simulink model "fwv_fulatti"  (R2021b)
settings: Solver=ode15s  StartTime=0.0  StopTime=10  FixedStep=0.01  MaxStep=0.01  RelTol=1e-3  AbsTol=1e-3  EnableMultiTasking=on
model workspace (MATLAB code in the model file):
  | p0=[0 0 0];
values from neighbouring files (symbols this model uses):
  A_D = 1.5    [main.m]    (also in param.m; params.m)
  A_L = 1.8    [main.m]    (also in param.m; params.m)
  c_bar = S/R    (= 0.0357142857143)    [main.m]    (also in param.m = 0.0251327412287; params.m)
  C_D0 = 0.45    [main.m]    (also in param.m; params.m)
  m = 2    [rbf_pid.m]
  r00 = double(int(f,[0,1]))    [main.m]    (also in param.m = 1; params.m = 0.933333333333)
  r11 = double(int(x*f,[0,1]))    [main.m]    (also in param.m = double(int(curv(x)*(x+1/9),0,1)); params.m = 0.481185185185)
  r22 = double(int(x^2*f,[0,1]))    [main.m]    (also in param.m = double(int(curv(x)*(x+1/9)^2,0,1)); params.m = 0.304750617284)
  r33 = double(int(x^3*f,[0,1]))    [main.m]    (also in param.m = double(int(curv(x)*(x+1/9)^3,0,1)); params.m = 0.218568691358)
  r_cp = Rw*r33/r22    [main.m]    (also in param.m; params.m = 0.10758076225)
  rho = 1.205    [main.m]    (also in param.m; params.m)
  Rw = 0.15    [main.m]    (also in param.m = 0.075; params.m)
  z00 = double(int(f^2,[0,1]))    [main.m]    (also in param.m = double(int(curv(x)^2,0,1)); params.m = 1.00177777778)
  z11 = double(int(x*f^2,[0,1]))    [main.m]    (also in param.m = double(int(curv(x)^2*(x+1/9),0,1)); params.m = 0.484918518519)
  z22 = double(int(x^2*f^2,[0,1]))    [main.m]    (also in param.m = double(int(curv(x)^2*(x+1/9)^2,0,1)); params.m = 0.28785382716)
  zrd = double(int(f^4,[0,1]))    [main.m]    (also in param.m = double(int(curv(x)^4,0,1)); params.m = 1.29333866667)
undefined symbols (not defined in the file or in its folder): X, Y, Z
libraries: sm_lib x57, nesl_utility x45, vrlib x3, slpidlib x2
(part 1 of 3)
settings Model: NumberOfSteps=10  PacingRate=1000  Creator=jeff  LastModifiedBy=jeff
settings SolverCC: AutoScaleAbsTol=off  ZeroCrossAlgorithm=Adaptive  SolverResetMethod=Robust
settings DataIOCC: LimitDataPoints=on  MaxDataPoints=10000  DSMLogging=off  InspectSignalLogs=on  SaveTime=off  ReturnWorkspaceOutputs=off
settings OptimizationCC: LifeSpan=inf
settings DebuggingCC: AllowSymbolicDim=off  SFUnexpectedBacktrackingDiag=warning  SFNoUnconditionalDefaultTransitionDiag=warning  SFExecutionAtInitializationDiag=none  SFMachineParentedDataDiag=warning  ArithmeticOperatorsInVariantConditions=warning
settings ModelReferenceCC: ModelReferenceMinAlgLoopOccurrences=on
settings SFSimCC: SimUseLocalCustomCode=off  CustomCodeUndefinedFunction=UseInterfaceOnly
settings RTWCC: RTWUseLocalCustomCode=off
settings CodeAppCC: StateflowObjectComments=on
settings GRTTargetCC: TargetLangStandard=C89/C90 (ANSI)
settings ConfigComp: CovMetricSettings=dw  CovSaveCumulativeToWorkspaceVar=on  CovSaveSingleToWorkspaceVar=on  CovExternalEMLEnable=off  CovSFcnEnable=off
settings SimscapeCC: SimscapeLogType=all  SimscapeLogSimulationStatistics=on  SimscapeLogDataHistory=10000
settings ExplorerConfigSet: InternalSimMechanicsExplorerSettings="<ExplorerConfiguration><canonicalview>default</canonicalview><AnimationSetting><BasePlaybackSpeed>1.0</BasePlaybackSpeed><PlaybackSpeedFactor>1.0</PlaybackSpeedFactor></AnimationSetting><TilePanel><TileInfo><Tiles Columns=\"2\" Count=\"4\" Rows=\"2\"><Column Weight=\"0.5\"/><Column Weight=\"0.5\"/><Row Weight=\"0.4982\"/><Row Weight=\"0.5018\"/><Tile Height=\"1\" Width=\"1\" X=\"0\" Y=\"0\"/><Tile Height=\"1\" Width=\"1\" X=\"0\" Y=\"1\"/><Tile Height=\"1\" Width=\"1\" X=\"1\" Y=\"0\"/><Tile Height=\"1\" Width=\"1\" X=\"1\" Y=\"1\"/></Tiles></TileInfo><SceneInfo><SceneViewer><BGColor><R>0.60000002384185791</R><G>0.60000002384185791</G><B>0.60000002384185791</B></BGColor><Camera><DoPerspective>off</DoPerspective><Position><X>1.52276591336431011e-07</X><Y>-15.7283506478538051</Y><Z>0.997276938595945239</Z></Position><Center><X>1.52276591336431011e-07</X><Y>8.81149515574719544e-08</Y><Z>0.997276938595945239</Z></Center><Up><X>0</X><Y>-0</Y><Z>1</Z></Up><ViewLimDist>1</ViewLimDist><YLim>4.13867069486404926</YLim><XLim>10.3000000000000007</XLim></Camera></SceneViewer><SceneViewer><BGColor><R>0.60000002384185791</R><G>0.60000002384185791</G><B>0.60000002384185791</B></BGColor><Camera><DoPerspective>off</DoPerspective><Position><X>1.52276591336431011e-07</X><Y>-4.72670020457144346e-07</Y><Z>14.1965844691727394</Z></Position><Center><X>1.52276591336431011e-07</X><Y>-4.72670020457144346e-07</Y><Z>0.997276770136494406</Z></Center><Up><X>0</X><Y>1</Y><Z>-0</Z></Up><ViewLimDist>1</ViewLimDist><YLim>10.3000000000000007</YLim><XLim>25.4425373134328368</XLim></Camera></SceneViewer><SceneViewer><BGColor><R>0.60000002384185791</R><G>0.60000002384185791</G><B>0.60000002384185791</B></BGColor><Camera><DoPerspective>off</DoPerspective><Position><X>15.7283506450403667</X><Y>-4.72670020457144346e-07</Y><Z>0.997277415433075021</Z></Position><Center><X>1.16597679067353965e-06</X><Y>-4.72670020457144346e-07</Y><Z>0.997277415433075021</Z></Center><Up><X>-0</X><Y>0</Y><Z>1</Z></Up><ViewLimDist>1</ViewLimDist><YLim>4.13867069486404926</YLim><XLim>10.3000000000000007</XLim></Camera></SceneViewer><SceneViewer><BGColor><R>0.60000002384185791</R><G>0.60000002384185791</G><B>0.60000002384185791</B></BGColor><Camera><DoPerspective>on</DoPerspective><Position><X>2.15185180954951205</X><Y>2.000061471445302</Y><Z>2.10008566610887026</Z></Position><Center><X>2.00185180954951214</X><Y>2.000061471445302</Y><Z>2.00008566610887017</Z></Center><Up><X>0</X><Y>-3.08148791101957736e-33</Y><Z>1</Z></Up><ViewLimDist>1</ViewLimDist><YLim>0.466307658154998583</YLim><XLim>1.15184951380078004</XLim></Camera></SceneViewer></SceneInfo></TilePanel><MechEditorPanel><Cameras><Camera><Id>Camera1</Id><Value><Name>Camera1</Name><NativeCamera><PositionTrackingFeature>FWV.camera.camera_Frame.R</PositionTrackingFeature><CenterTrackingFeature>FWV.camera.C</CenterTrackingFeature><UpVectorTrackingFeature>FWV.camera.C</UpVectorTrackingFeature><CenterTrackingOrigin>on</CenterTrackingOrigin><UpVectorTrackingDirection>+Z</UpVectorTrackingDirection></NativeCamera></Value></Camera></Cameras><GfxPanelCameraMap><MapElement CameraMLId=\"Camera1\" GfxPanelIndex=\"3\"/></GfxPanelCameraMap><VideoCreator><PlaybackSpeedRatio>1.0</PlaybackSpeedRatio><FrameRate>30</FrameRate><VideoFormat>Motion JPEG AVI</VideoFormat><FrameSize>auto</FrameSize></VideoCreator></MechEditorPanel></ExplorerConfiguration>"

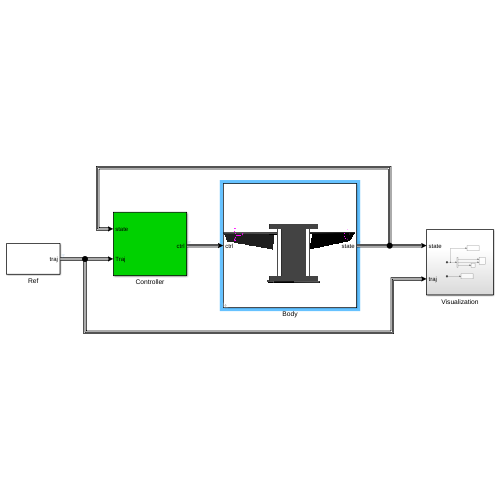
[thumbnail: Simulink's stored preview of the top-level diagram]
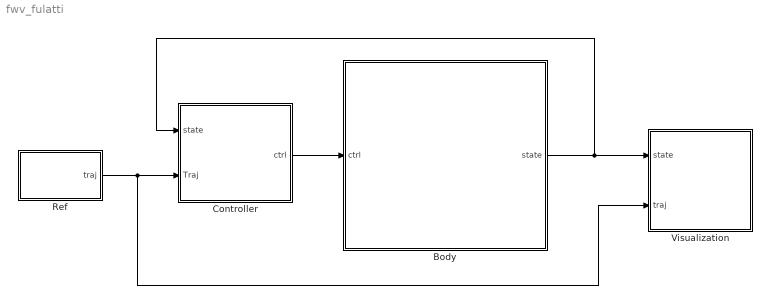
== system fwv_fulatti ==
  Body : Subsystem  mask{rho_w=900, m_t=20, stif_stk=0, stif_rot=5e-3, damp_rot=0, stif_m=1e2, damp_m=1e2, z0=0, p0=0, q0=0, r0=0}
      mask prompts: z0 "initial height"; p0 "initial roll(deg)"; q0 "initial pitch(deg)"; r0 "initial yaw(deg)"
      mask Display: image('Images/fwv.png');
  Controller : Subsystem
  Ref : Subsystem
  Visualization : Subsystem
  wires:
  Ref/1(traj) -> Visualization/2(traj), Controller/2(Traj)
  Controller/1(ctrl) -> Body/1(ctrl)
  Body/1(state) -> Controller/1(state), Visualization/1(state)

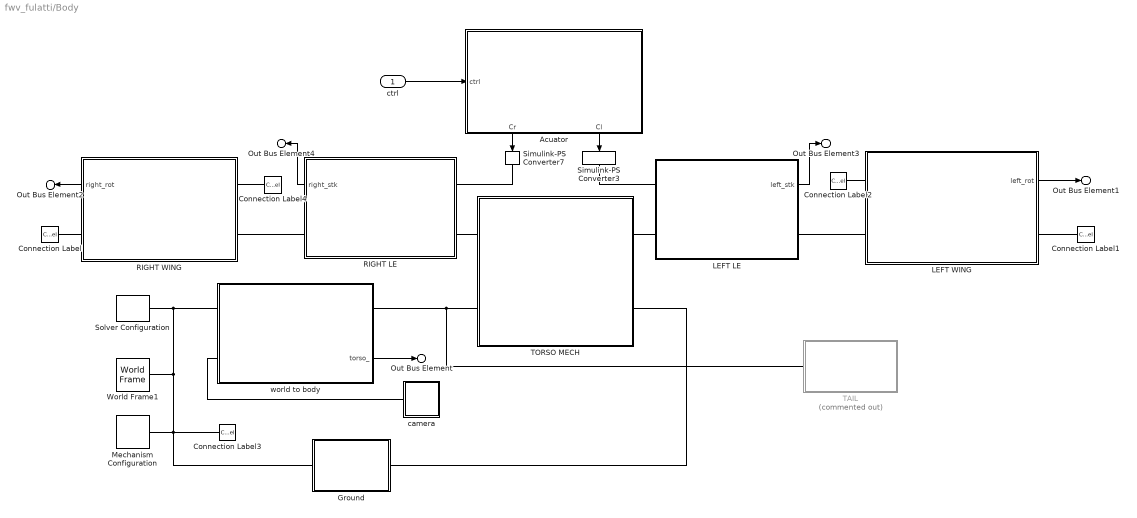
== system fwv_fulatti/Body ==
  ctrl : Inport
  Acuator : Subsystem
      settings: PortSchema="{\"entries\":[{\"content\":{\"sides\":[{\"content\":{\"connectorIds\":[\"In1\"]},\"type\":\"ConnectorPlacement.EquallySpacedRectSide\",\"uuid\":\"db46f0ff-2b35-4735-b2ba-99ebad500531\"},{\"content\":{\"connectorIds\":[],\"side\":\"RIGHT\"},\"type\":\"ConnectorPlacement.EquallySpacedRectSide\",\"uuid\":\"a05d2a9d-5b8e-445a-bb52-abca9ea78047\"},{\"content\":{\"connectorIds\":[],\"side\":\"TOP\"},\"type\":\"ConnectorPlacement.EquallySpacedRectSide\",\"uuid\":\"a9e07a0b-59af-45c6-89e8-be07490c71bb\"},{\"content\":{\"connectorIds\":[\"Out1\",\"Out2\"],\"side\":\"BOTTOM\"},\"type\":\"ConnectorPlacement.EquallySpacedRectSide\",\"uuid\":\"69a70806-995a-45b1-874e-667630f2a15c\"}]},\"type\":\"ConnectorPlacement.EquallySpacedConnector\",\"uuid\":\"cc8e5811-56fa-45cd-8c97-474062c30ea3\"}],\"packageUris\":[\"http://schema.mathworks.com/mf0/Connector/R2020b\"],\"version\":\"1.0\"}"
  Connection Label : ConnectionLabel  Label=CP_R
  Connection Label1 : ConnectionLabel  Label=CP_L
  Connection Label2 : ConnectionLabel  Label=W
  Connection Label3 : ConnectionLabel  Label=W
  Connection Label4 : ConnectionLabel  Label=W
  Ground : Subsystem
  LEFT LE : Subsystem
      mask Display: image('Images/lle.png'); % Use "Edit Image" on toolstrip to change.
  LEFT WING : Subsystem
      mask Display: image('Images/lwing.png'); % Use "Edit Image" on toolstrip to change.
  Mechanism Configuration : sm_lib/Utilities/Mechanism Configuration  UniformGravity=Constant  GravityVector=[0 0 -9.80665]  GravityUnits=m/s^2  LinearizationDelta=0.001  JointModeTransitionNonlinearIterations=2
  RIGHT LE : Subsystem
      settings: PortSchema="{\"entries\":[{\"content\":{\"sides\":[{\"content\":{\"connectorIds\":[\"Out1\",\"LConn1\"]},\"type\":\"ConnectorPlacement.EquallySpacedRectSide\",\"uuid\":\"e80f0529-82a8-4e91-8f70-1f5fff48efb0\"},{\"content\":{\"connectorIds\":[\"RConn1\",\"RConn2\"],\"side\":\"RIGHT\"},\"type\":\"ConnectorPlacement.EquallySpacedRectSide\",\"uuid\":\"c7e3ee7d-7bee-46da-b210-768e5832b89d\"},{\"content\":{\"connectorIds\":[],\"side\":\"TOP\"},\"type\":\"ConnectorPlacement.EquallySpacedRectSide\",\"uuid\":\"680cbd67-40e5-4a58-a196-f2062cf587c7\"}]},\"type\":\"ConnectorPlacement.EquallySpacedConnector\",\"uuid\":\"7cb1a5ec-7352-40bf-9e6c-a29cba360f94\"}],\"packageUris\":[\"http://schema.mathworks.com/mf0/Connector/R2020b\"],\"version\":\"1.0\"}"
      mask Display: image('Images/rle.png'); % Use "Edit Image" on toolstrip to change.
  RIGHT WING : Subsystem
      mask Display: image('Images/rwing.png'); % Use "Edit Image" on toolstrip to change.
  Simulink-PS Converter3 : nesl_utility/Simulink-PS Converter  PhysicalDomain=network_engine_domain  SubClassName=ps_input  LeftPortType=input  RightPortType=output  PseudoPeriodic=off  Frequencies=[]  NoiseDistribution=none  NoiseParameters=[]  Unit=1  AffineConversion=off  FilteringAndDerivatives=filter  SimscapeFilterOrder=2  InputFilterTimeConstant=0.001  UdotUserProvided=2
      settings: SourceProductBaseCode=PW,SS
  Simulink-PS Converter7 : nesl_utility/Simulink-PS Converter  PhysicalDomain=network_engine_domain  SubClassName=ps_input  LeftPortType=input  RightPortType=output  PseudoPeriodic=off  Frequencies=[]  NoiseDistribution=none  NoiseParameters=[]  Unit=1  AffineConversion=off  FilteringAndDerivatives=filter  SimscapeFilterOrder=2  InputFilterTimeConstant=0.001  UdotUserProvided=0
      settings: SourceProductBaseCode=PW,SS
  Solver Configuration : nesl_utility/Solver Configuration  PhysicalDomain=network_engine_domain  SubClassName=solver  LeftPortType=input  RightPortType=generic  Tones=[]  Harmonics=[]  SimulateNoise=off  Profile=off  UseLocalSampling=off  EnableSwitchedLinearOptims=on  FrequencyDomain=off  UseCCode=off  RelTol=0.001  AbsTol=1e-06  MinStep=1e-09  ToWorkspace=off  RevertToSquareIcSolve=off  NumHomotopyIterations=100  PhasorMode=off  PhasorModeNumHarmonics=1  DoDC=off  ResidualTolerance=1e-09  UseLocalSolver=off  LocalSolverChoice=NE_BACKWARD_EULER_ADVANCER  LocalSolverSampleTime=0.001  DoFixedCost=off  MaxNonlinIter=3  MaxModeIter=2  ComputeImpulses=off  ImpulseIterations=2  LinearAlgebra=Sparse  EquationFormulation=NE_TIME_EF  DelaysMemoryBudget=1024  AutomaticFiltering=on  FilteringTimeConstant=0.001  PartitionStorageMethod=AS_NEEDED  PartitionMemoryBudget=1024  PartitionMethod=FAST
      settings: SourceProductBaseCode=PW,SS
  TAIL : Subsystem  Commented=on
  TORSO MECH : Subsystem  mask{mu0=0, mu1=0}
      mask Display: image('Images/fuselage.png'); % Use "Edit Image" on toolstrip to change.
  World Frame1 : sm_lib/Frames and Transforms/World Frame
  camera : Subsystem
  world to body : Subsystem
      settings: PortSchema="{\"entries\":[{\"content\":{\"sides\":[{\"content\":{\"connectorIds\":[\"LConn1\",\"LConn2\"]},\"type\":\"ConnectorPlacement.EquallySpacedRectSide\",\"uuid\":\"67e08b7d-27a7-478e-aa2b-0a29cfb8c4ba\"},{\"content\":{\"connectorIds\":[\"RConn1\",\"Out1\"],\"side\":\"RIGHT\"},\"type\":\"ConnectorPlacement.EquallySpacedRectSide\",\"uuid\":\"af848fd7-c404-4734-a34f-7cffff1411b1\"},{\"content\":{\"connectorIds\":[],\"side\":\"TOP\"},\"type\":\"ConnectorPlacement.EquallySpacedRectSide\",\"uuid\":\"40c86437-2469-4d2e-8b61-7b3eee85e893\"}]},\"type\":\"ConnectorPlacement.EquallySpacedConnector\",\"uuid\":\"cd10b607-3f85-4cd2-a6c3-0d07bf2597bd\"}],\"packageUris\":[\"http://schema.mathworks.com/mf0/Connector/R2020b\"],\"version\":\"1.0\"}"
  Out Bus Element : Outport  PortName=state  Element=pose
  Out Bus Element3 : Outport  PortName=state  Element=left_stk
  Out Bus Element1 : Outport  PortName=state  Element=left_rot
  Out Bus Element4 : Outport  PortName=state  Element=right_stk
  Out Bus Element2 : Outport  PortName=state  Element=right_rot
  wires:
  LEFT WING/1(left_rot) -> Out Bus Element1/1
  RIGHT WING/1(right_rot) -> Out Bus Element2/1
  world to body/1(torso_) -> Out Bus Element/1
  Acuator/2(Cl) -> Simulink-PS Converter3/1
  Acuator/1(Cr) -> Simulink-PS Converter7/1
  ctrl/1 -> Acuator/1(ctrl)
  LEFT LE/1(left_stk) -> Out Bus Element3/1
  RIGHT LE/1(right_stk) -> Out Bus Element4/1
  connections:
  LEFT LE/LConn2 -- TORSO MECH/RConn1
  TORSO MECH/LConn1 -- RIGHT LE/RConn2
  Simulink-PS Converter7/RConn1 -- RIGHT LE/RConn1
  Mechanism Configuration/RConn1 -- Connection Label3/LConn1 -- Ground/LConn1 -- world to body/LConn1 -- Solver Configuration/RConn1 -- World Frame1/RConn1
  world to body/RConn1 -- TAIL/LConn1 -- TORSO MECH/LConn2
  camera/LConn1 -- world to body/LConn2
  Ground/RConn1 -- TORSO MECH/RConn2
  Connection Label/LConn1 -- RIGHT WING/RConn1
  LEFT WING/RConn1 -- Connection Label1/LConn1
  Simulink-PS Converter3/RConn1 -- LEFT LE/LConn1
  LEFT WING/LConn2 -- LEFT LE/RConn1
  RIGHT WING/LConn2 -- RIGHT LE/LConn1
  Connection Label2/LConn1 -- LEFT WING/LConn1
  Connection Label4/LConn1 -- RIGHT WING/LConn1

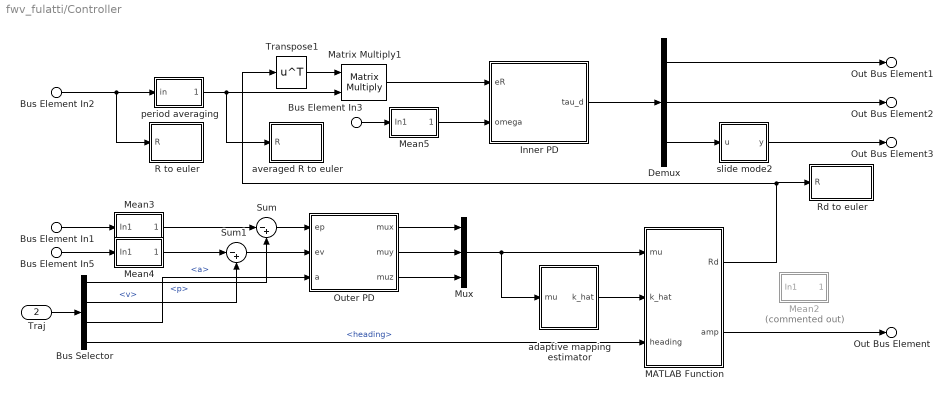
== system fwv_fulatti/Controller ==
  Bus Element In1 : Inport  PortName=state  Element=pose.p
  Bus Element In2 : Inport  PortName=state  Element=pose.R
  Bus Element In3 : Inport  PortName=state  Element=pose.w
  Bus Element In5 : Inport  PortName=state  Element=pose.v
  Traj : Inport  Port=2
  Bus Selector : BusSelector  OutputSignals=p,v,a,heading
  Demux : Demux  Outputs=3
  Inner PD : Subsystem
  MATLAB Function : MATLAB Function  TreatAsAtomicUnit=on
  Matrix Multiply1 : Product  Multiplication=Matrix(*)
  Mean2 : Subsystem  Commented=on
  Mean3 : Subsystem
  Mean4 : Subsystem
  Mean5 : Subsystem
  Mux : Mux  Inputs=3
  Outer PD : Subsystem
  R to euler : Subsystem
  Rd to euler : Subsystem
      settings: PortSchema="{\"entries\":[{\"content\":{\"sides\":[{\"content\":{\"connectorIds\":[]},\"type\":\"ConnectorPlacement.EquallySpacedRectSide\",\"uuid\":\"93de112d-0217-40d7-a336-17ea7cc4ed84\"},{\"content\":{\"connectorIds\":[\"In1\"],\"side\":\"RIGHT\"},\"type\":\"ConnectorPlacement.EquallySpacedRectSide\",\"uuid\":\"0b203bc8-f5c1-4f94-b862-0e0b0c3261f7\"},{\"content\":{\"connectorIds\":[],\"side\":\"TOP\"},\"type\":\"ConnectorPlacement.EquallySpacedRectSide\",\"uuid\":\"1be19d4c-6517-470f-aabd-96bb4bcaed3d\"}]},\"type\":\"ConnectorPlacement.EquallySpacedConnector\",\"uuid\":\"f5fc68b0-193c-43e6-a8c2-776496b24de9\"}],\"packageUris\":[\"http://schema.mathworks.com/mf0/Connector/R2020b\"],\"version\":\"1.0\"}"
  Sum : Sum  Inputs=|-+
  Sum1 : Sum  Inputs=|-+
  Transpose1 : Math  Operator=transpose  SaturateOnIntegerOverflow=on
  adaptive mapping estimator : Subsystem
  averaged R to euler : Subsystem
  period averaging : Subsystem
  slide mode2 : MATLAB Function  TreatAsAtomicUnit=on
  Out Bus Element : Outport  PortName=ctrl  Element=amp_mean
  Out Bus Element1 : Outport  PortName=ctrl  Element=amp_diff
  Out Bus Element2 : Outport  PortName=ctrl  Element=bias
  Out Bus Element3 : Outport  PortName=ctrl  Element=offset
  wires:
  Traj/1 -> Bus Selector/1
  Bus Selector/1 -> Sum/2  "<p>"
  Inner PD/1(tau_d) -> Demux/1
  Transpose1/1 -> Matrix Multiply1/1
  Bus Selector/2 -> Sum1/2  "<v>"
  Bus Selector/3 -> Outer PD/3(a)  "<a>"
  Bus Element In2/1 -> R to euler/1(R), period averaging/1(in)
  Bus Selector/4 -> MATLAB Function/3(heading)  "<heading>"
  Sum/1 -> Outer PD/1(ep)
  Sum1/1 -> Outer PD/2(ev)
  Outer PD/3(muz) -> Mux/3
  Mux/1 -> MATLAB Function/1(mu), adaptive mapping estimator/1(mu)
  Matrix Multiply1/1 -> Inner PD/1(eR)
  Demux/3 -> slide mode2/1(u)
  MATLAB Function/1(Rd) -> Transpose1/1, Rd to euler/1(R)
  Bus Element In1/1 -> Mean3/1(In1)
  Bus Element In5/1 -> Mean4/1(In1)
  Mean3/1(Mean1) -> Sum/1
  Mean4/1(Mean1) -> Sum1/1
  Bus Element In3/1 -> Mean5/1(In1)
  Mean5/1(Mean1) -> Inner PD/2(omega)
  MATLAB Function/2(amp) -> Out Bus Element/1
  period averaging/1(Mean1) -> averaged R to euler/1(R), Matrix Multiply1/2
  adaptive mapping estimator/1(k_hat) -> MATLAB Function/2(k_hat)
  Outer PD/1(mux) -> Mux/1
  Outer PD/2(muy) -> Mux/2
  Demux/1 -> Out Bus Element1/1
  Demux/2 -> Out Bus Element2/1
  slide mode2/1(y) -> Out Bus Element3/1

== system fwv_fulatti/Ref ==
  Bus Creator : BusCreator  Inputs=4
  Clock : Clock
  p,pdot,pddot : MATLAB Function  TreatAsAtomicUnit=on
  traj : Outport
  wires:
  Bus Creator/1 -> traj/1
  p,pdot,pddot/3(v) -> Bus Creator/3  "v"
  p,pdot,pddot/4(a) -> Bus Creator/4  "a"
  Clock/1 -> p,pdot,pddot/1(t)
  p,pdot,pddot/1(p) -> Bus Creator/1  "p"
  p,pdot,pddot/2(heading) -> Bus Creator/2

== system fwv_fulatti/Visualization ==
  Bus Element In1 : Inport  PortName=state  Element=pose.p
  Bus Element In : Inport  Port=2  PortName=traj  Element=p
  Demux : Demux  Outputs=3
  Terminator : Terminator
  To Workspace : ToWorkspace  VariableName=p  SampleTime=-1
      settings: Save2DSignal=2-D array (concatenate along first dimension)
  To Workspace1 : ToWorkspace  VariableName=pd  SampleTime=-1
      settings: Save2DSignal=2-D array (concatenate along first dimension)
  XY Graph : Record  FileSettingsInternal="{\"entries\":[{\"content\":{\"excelSettings\":{\"content\":{},\"type\":\"Streamout.ExcelSettings\"}},\"type\":\"Streamout.FileSettingStorage\",\"uuid\":\"cf1958ac-8bfe-45ed-8e34-609005fdbf73\"}],\"packageUris\":[\"http://schema.mathworks.com/mf0/streamout_blocks/R2020a\"],\"version\":\"1.0\"}"  Layout=[1 1]  SignalsInternal="{\"entries\":[{\"content\":{\"signals\":[{\"content\":{\"blockPath\":[\"fwv_fulatti/Visualization/XY Graph\"],\"channel\":[],\"dimensions\":[1],\"domain\":\"fwv_fulatti/Visualization/XY Graph\",\"lineColor\":\"#fe330a\",\"plots\":[],\"port\":1,\"sid\":[\"\"],\"signalID\":154858,\"signalName\":\"Demux:1\"},\"type\":\"RecordBlkView.Signal\",\"uuid\":\"53ba67ad-0e88-436d-a209-32f50bd88dfe\"},{\"content\":{\"blockPath\":[\"fwv_fulatti/Visualization/XY Graph\"],\"channel\":[],\"dimensions\":[1],\"domain\":\"fwv_fulatti/Visualization/XY Graph\",\"lineColor\":\"#22b573\",\"plots\":[],\"port\":2,\"sid\":[\"\"],\"signalID\":154862,\"signalName\":\"Demux:2\"},\"type\":\"RecordBlkView.Signal\",\"uuid\":\"95253e4f-1692-44e6-a8ad-d105dc3e908e\"}]},\"type\":\"RecordBlkView.InputSignals\",\"uuid\":\"3e219576-be3c-4ed1-8d49-ea9d7e7a7c36\"}],\"packageUris\":[\"http://schema.mathworks.com/mf0/streamout_blocks/R2020a\"],\"version\":\"1.0\"}"  VisualizationBindings="{\"xyplotplugin\":{\"info\":[{\"series\":[],\"subplotID\":1}]}}"  CompatibilityTag=XY  st=-1
  wires:
  Bus Element In1/1 -> To Workspace/1, Demux/1
  Demux/3 -> Terminator/1
  Demux/1 -> XY Graph/1
  Demux/2 -> XY Graph/2
  Bus Element In/1 -> To Workspace1/1

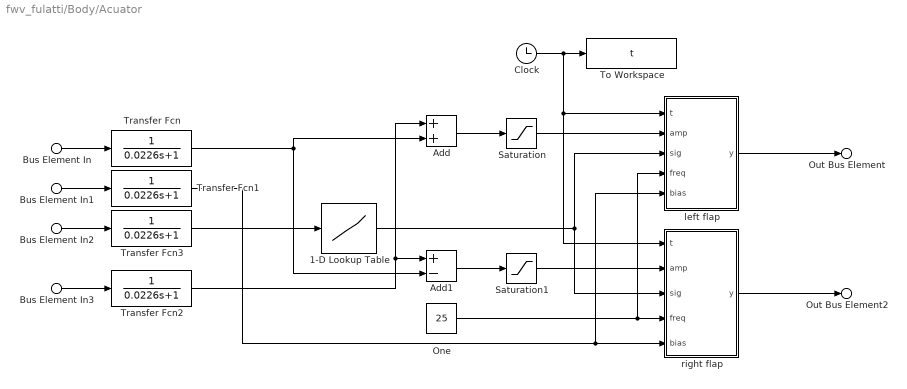
== system fwv_fulatti/Body/Acuator ==
  Bus Element In3 : Inport  PortName=ctrl  Element=amp_mean
  Bus Element In : Inport  PortName=ctrl  Element=amp_diff
  Bus Element In1 : Inport  PortName=ctrl  Element=bias
  Bus Element In2 : Inport  PortName=ctrl  Element=offset
  " left flap" : MATLAB Function  TreatAsAtomicUnit=on
  " right flap" : MATLAB Function  TreatAsAtomicUnit=on
  1-D Lookup Table : Lookup_n-D  NumberOfTableDimensions=1  BreakpointsForDimension1=[-1:1]  Table=1.0./(1+exp(-10*[-1:1]))  InternalRulePriority=Speed  RndMeth=Simplest  InputSameDT=on
  Add : Sum
  Add1 : Sum  Inputs=+-
  Clock : Clock
  One : Constant  Value=25  OutDataTypeStr=Inherit: Inherit via back propagation
  Saturation : Saturate  UpperLimit=pi/2  LowerLimit=0  ZeroCross=off
  Saturation1 : Saturate  UpperLimit=pi/2  LowerLimit=0  ZeroCross=off
  To Workspace : ToWorkspace  VariableName=t  SampleTime=-1
  Transfer Fcn{,1..3} (4 alike) : TransferFcn  Denominator=[0.0226 1]
  Out Bus Element2 : Outport  PortName=Cr  Element=stroke
  Out Bus Element : Outport  Port=2  PortName=Cl  Element=stroke
  wires:
  Add1/1 -> Saturation1/1
  " left flap"/1(y) -> Out Bus Element/1
  One/1 -> " left flap"/4(freq), " right flap"/4(freq)
  " right flap"/1(y) -> Out Bus Element2/1
  Add/1 -> Saturation/1
  Saturation/1 -> " left flap"/2(amp)
  Clock/1 -> " right flap"/1(t), " left flap"/1(t), To Workspace/1
  Saturation1/1 -> " right flap"/2(amp)
  Transfer Fcn2/1 -> Add/1, Add1/1
  Transfer Fcn/1 -> Add1/2, Add/2
  Bus Element In/1 -> Transfer Fcn/1
  Bus Element In1/1 -> Transfer Fcn1/1
  Bus Element In2/1 -> Transfer Fcn3/1
  Bus Element In3/1 -> Transfer Fcn2/1
  Transfer Fcn1/1 -> " left flap"/5(bias), " right flap"/5(bias)
  Transfer Fcn3/1 -> 1-D Lookup Table/1
  1-D Lookup Table/1 -> " right flap"/3(sig), " left flap"/3(sig)

== system fwv_fulatti/Body/Ground ==
  Cylindrical Solid : sm_lib/Body Elements/Cylindrical Solid  GraphicAmbientColor=[0.15 0.15 0.15 1.0]  BasedOnType=Mass  CenterOfMass=[0 0 0]  CenterOfMassUnits=m  GraphicDiffuseColor=[1.0 0.2 0.4]  CylinderLength=1  CylinderLengthUnits=mm  CylinderRadius=10  CylinderRadiusUnits=m  Density=1000  DensityUnits=kg/m^3  DoExposeReferenceFrame=off  GraphicEmissiveColor=[0.0 0.0 0.0 1.0]  ExportEntireGeometry=on  SerializedFrames=<Frames><Frame><Id>Frame1</Id><Value><Name>F1</Name><Origin><Source>GeometricFeature</Source><FeatureName>top surface</FeatureName></Origin><PrimaryAxis><DefinedDirection>+Z</DefinedDirection><Source>ReferenceFrame</Source><SourceDirection>+Z</SourceDirection><FeatureName></FeatureName></PrimaryAxis><SecondaryAxis><DefinedDirection>+X</DefinedDirection><Source>ReferenceFrame</Source><SourceDirection>+X</SourceDirection><FeatureName></FeatureName></SecondaryAxis></Value></Frame></Frames>  MarkerShape=Sphere  MarkerSize=10  GraphicType=FromGeometry  InertiaType=Custom  Mass=0  MassUnits=kg  MomentsOfInertia=[1 1 1]  MomentsOfInertiaUnits=kg*m^2  GraphicOpacity=1.0  ProductsOfInertia=[0 0 0]  ProductsOfInertiaUnits=kg*m^2  GraphicShininess=75  GraphicSpecularColor=[0.5 0.5 0.5 1.0]  GraphicVisPropType=SimpleVisualProperties
  Rigid Transform : sm_lib/Frames and Transforms/Rigid Transform  TranslationMethod=StandardAxis  TranslationStandardOffset=6  TranslationLengthUnit=cm  TranslationStandardAxis=-Z  TranslationCartesianOffset=[0 0 0]  TranslationROffset=0  TranslationROffsetUnits=m  TranslationZOffset=0  TranslationZOffsetUnits=m  TranslationThetaOffset=0  TranslationThetaOffsetUnits=deg  RotationMethod=None  RotationAngleUnits=deg  RotationStandardAxis=+Z  RotationAngle=0.0  RotationArbitraryAxis=[0 0 1]  FollAlignAxisA=+X  BaseAlignAxisA=+Y  FollAlignAxisB=+Y  BaseAlignAxisB=+Z  RotationSequenceAxes=FollowerAxes  RotationSequence=XYX  RotationSequenceAngles=[0 0 0]  RotationSequenceAnglesUnits=deg  RotationMatrix=[1 0 0; 0 1 0; 0 0 1]
  W : PMIOPort  Side=Left
  G : PMIOPort  Port=2  Side=Right
  connections:
  G/RConn1 -- Cylindrical Solid/RConn1
  Rigid Transform/LConn1 -- W/RConn1
  Rigid Transform/RConn1 -- Cylindrical Solid/LConn1

== system fwv_fulatti/Body/LEFT LE ==
  Left LE1 : sm_lib/Body Elements/File Solid  ExtGeomFileName=meshes/left_LE.step  UnitType=FromFile  ExtGeomFileUnits=m  StepReaderType=HEX  ExportConvexHullGeometry=off  InertiaType=Custom  Mass=1  MassUnits=g  CenterOfMass=[0 0.0453 0.0239]  CenterOfMassUnits=m  MomentsOfInertia=[3.2e-06, 7.22e-07, 2.48e-06]  MomentsOfInertiaUnits=kg*m^2  ProductsOfInertia=[-7.2975e-07 0 0]  ProductsOfInertiaUnits=kg*m^2  BasedOnType=Mass  Density=800  DensityUnits=kg/m^3  DoExposeReferenceFrame=on  SerializedFrames=<Frames/>  GraphicType=FromGeometry  MarkerShape=Sphere  MarkerSize=10  GraphicVisPropType=SimpleVisualProperties  GraphicDiffuseColor=[0.5 0.5 0.5]  GraphicSpecularColor=[0.5 0.5 0.5 1.0]  GraphicAmbientColor=[0.15 0.15 0.15 1.0]  GraphicEmissiveColor=[0.0 0.0 0.0 1.0]  GraphicShininess=75  GraphicOpacity=1.0
  PS-Simulink Converter13 : nesl_utility/PS-Simulink Converter  PhysicalDomain=network_engine_domain  SubClassName=ps_output  LeftPortType=input  RightPortType=output  PseudoPeriodic=off  Frequencies=[]  Unit=inherit  AffineConversion=off
      settings: SourceProductBaseCode=PW,SS
  PS-Simulink Converter17 : nesl_utility/PS-Simulink Converter  PhysicalDomain=network_engine_domain  SubClassName=ps_output  LeftPortType=input  RightPortType=output  PseudoPeriodic=off  Frequencies=[]  Unit=inherit  AffineConversion=off
      settings: SourceProductBaseCode=PW,SS
  Stroke Joint : sm_lib/Joints/Revolute Joint  JointMode=Normal  SenseConstraintForce=off  SenseConstraintForceX=off  SenseConstraintForceY=off  SenseConstraintForceZ=off  SenseConstraintTorque=off  SenseConstraintTorqueX=off  SenseConstraintTorqueY=off  SenseConstraintTorqueZ=off  SenseTotalForce=off  SenseTotalForceX=off  SenseTotalForceY=off  SenseTotalForceZ=off  SenseTotalTorque=off  SenseTotalTorqueX=off  SenseTotalTorqueY=off  SenseTotalTorqueZ=off  CompositeWrenchDir=FollowerOnBase  CompositeWrenchFrame=BaseFrame  EquilibriumPosition=0  EquilibriumPositionUnits=deg  SpringStiffness=stif_stk  SpringStiffnessUnits=N*m/rad  DampingCoefficient=0  DampingCoefficientUnits=N*m/(rad/s)  TorqueActuationMode=ComputedTorque  MotionActuationMode=InputMotion  SensePosition=on  SenseVelocity=on  SenseAcceleration=off  SenseTorqueForce=off  SenseLowerLimitTorqueForce=off  SenseUpperLimitTorqueForce=off  LowerLimitSpecify=on  LowerLimitBound=-90  LowerLimitBoundUnits=deg  LowerLimitStiffness=1e6  LowerLimitStiffnessUnits=N*m/rad  LowerLimitDamping=1e3  LowerLimitDampingUnits=N*m/(rad/s)  LowerLimitTransitionRegionWidth=0.1  LowerLimitTransitionRegionWidthUnits=deg  UpperLimitSpecify=on  UpperLimitBound=90  UpperLimitBoundUnits=deg  UpperLimitStiffness=1e6  UpperLimitStiffnessUnits=N*m/rad  UpperLimitDamping=1e3  UpperLimitDampingUnits=N*m/(rad/s)  UpperLimitTransitionRegionWidth=0.1  UpperLimitTransitionRegionWidthUnits=deg  PositionTargetSpecify=off  PositionTargetPriority=High  PositionTargetValue=-30  PositionTargetValueUnits=deg  VelocityTargetSpecify=off  VelocityTargetPriority=High  VelocityTargetValue=0  VelocityTargetValueUnits=deg/s
  left Shoulder : sm_lib/Frames and Transforms/Rigid Transform  TranslationMethod=Cartesian  TranslationStandardOffset=0  TranslationLengthUnit=cm  TranslationStandardAxis=+Z  TranslationCartesianOffset=[0 1 4]  TranslationROffset=0  TranslationROffsetUnits=m  TranslationZOffset=0  TranslationZOffsetUnits=m  TranslationThetaOffset=0  TranslationThetaOffsetUnits=deg  RotationMethod=StandardAxis  RotationAngleUnits=deg  RotationStandardAxis=+X  RotationAngle=-90  RotationArbitraryAxis=[0 0 1]  FollAlignAxisA=+X  BaseAlignAxisA=+Y  FollAlignAxisB=+Y  BaseAlignAxisB=+Z  RotationSequenceAxes=FollowerAxes  RotationSequence=XYX  RotationSequenceAngles=[0 0 0]  RotationSequenceAnglesUnits=deg  RotationMatrix=[0 1 0; 0 0 1; 1 0 0]
  t of Left Stroke : PMIOPort  Side=Left
  LT : PMIOPort  Port=2  Side=Left
  WT : PMIOPort  Port=3  Side=Right
  Out Bus Element5 : Outport  PortName=left_stk  Element=q
  Out Bus Element6 : Outport  PortName=left_stk  Element=w
  wires:
  PS-Simulink Converter17/1 -> [psi_dot_l]
  PS-Simulink Converter13/1 -> [psi_l]
  [psi_l] -> Out Bus Element5/1
  [psi_dot_l] -> Out Bus Element6/1
  connections:
  Stroke Joint/RConn3 -- PS-Simulink Converter17/LConn1
  Stroke Joint/RConn2 -- PS-Simulink Converter13/LConn1
  Stroke Joint/LConn1 -- LT/RConn1
  Left LE1/RConn1 -- left Shoulder/LConn1 -- Stroke Joint/RConn1
  Stroke Joint/LConn2 -- t of Left Stroke/RConn1
  WT/RConn1 -- left Shoulder/RConn1

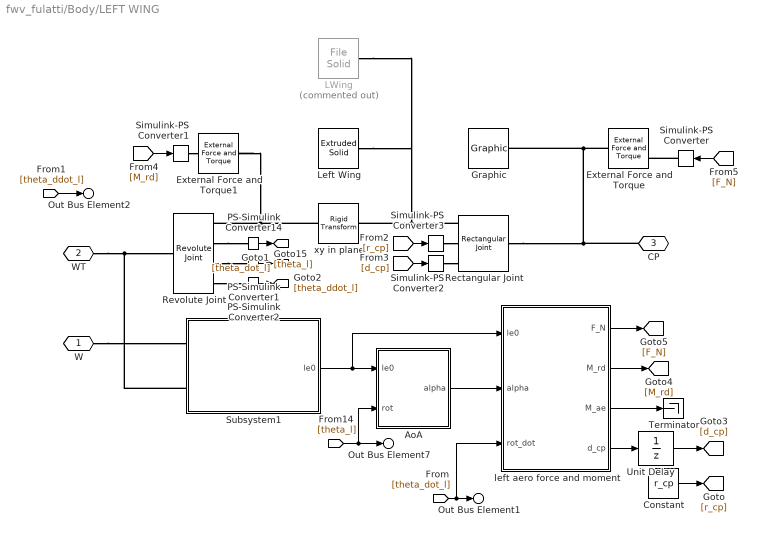
== system fwv_fulatti/Body/LEFT WING ==
  AoA : MATLAB Function  TreatAsAtomicUnit=on
  Constant : Constant  Value=r_cp
  External Force and Torque : sm_lib/Forces and Torques/External Force and Torque  ForceResolutionFrame=AttachedFrame  EnableForceX=off  EnableForceY=on  EnableForceZ=on  EnableForce=off  TorqueResolutionFrame=AttachedFrame  EnableTorqueX=off  EnableTorqueY=off  EnableTorqueZ=off  EnableTorque=off
  External Force and Torque1 : sm_lib/Forces and Torques/External Force and Torque  ForceResolutionFrame=AttachedFrame  EnableForceX=off  EnableForceY=off  EnableForceZ=off  EnableForce=off  TorqueResolutionFrame=AttachedFrame  EnableTorqueX=off  EnableTorqueY=off  EnableTorqueZ=on  EnableTorque=off
  Graphic : sm_lib/Body Elements/Graphic  GraphicType=Marker  MarkerShape=Frame  MarkerSize=20  GraphicVisPropType=SimpleVisualProperties  GraphicDiffuseColor=[1 0 1]  GraphicSpecularColor=[0.5 0.5 0.5 1.0]  GraphicAmbientColor=[0.15 0.15 0.15 1.0]  GraphicEmissiveColor=[0.0 0.0 0.0 1.0]  GraphicShininess=75  GraphicOpacity=1.0
  LWing : sm_lib/Body Elements/File Solid  Commented=on  ExtGeomFileName=meshes/left_wing.stl  UnitType=Custom  ExtGeomFileUnits=mm  StepReaderType=HEX  ExportConvexHullGeometry=off  InertiaType=CalculateFromGeometry  Mass=1  MassUnits=kg  CenterOfMass=[0 0 0]  CenterOfMassUnits=m  MomentsOfInertia=[1 1 1]  MomentsOfInertiaUnits=kg*m^2  ProductsOfInertia=[0 0 0]  ProductsOfInertiaUnits=kg*m^2  BasedOnType=Density  Density=rho_w  DensityUnits=kg/m^3  DoExposeReferenceFrame=on  SerializedFrames=<Frames/>  GraphicType=FromGeometry  MarkerShape=Sphere  MarkerSize=10  GraphicVisPropType=SimpleVisualProperties  GraphicDiffuseColor=[0.5 0.5 0.5]  GraphicSpecularColor=[0.5 0.5 0.5 1.0]  GraphicAmbientColor=[0.15 0.15 0.15 1.0]  GraphicEmissiveColor=[0.0 0.0 0.0 1.0]  GraphicShininess=75  GraphicOpacity=1.0
  Left Wing : sm_lib/Body Elements/Extruded Solid  GraphicAmbientColor=[0.15 0.15 0.15 1.0]  BasedOnType=Density  CenterOfMass=[0 0 0]  CenterOfMassUnits=m  GraphicDiffuseColor=[0.5 0.5 0.5]  ExportConvexHullGeometry=off  ExtrusionCrossSection=[0 0; 20 -50; 140 -25; 140 0]  ExtrusionCrossSectionUnits=mm  Density=rho_w  DensityUnits=kg/m^3  DoExposeReferenceFrame=on  GraphicEmissiveColor=[0.0 0.0 0.0 1.0]  ExportEntireGeometry=off  ExtrusionLength=0.1  ExtrusionLengthUnits=mm  ExtrusionType=General  SerializedFrames=<Frames/>  MarkerShape=Sphere  MarkerSize=10  GraphicType=FromGeometry  InertiaType=CalculateFromGeometry  Mass=1  MassUnits=kg  MomentsOfInertia=[1 1 1]  MomentsOfInertiaUnits=kg*m^2  PolygonNumSides=3  GraphicOpacity=1.0  PolygonOuterRadius=1  PolygonOuterRadiusUnits=m  ProductsOfInertia=[0 0 0]  ProductsOfInertiaUnits=kg*m^2  GraphicShininess=75  GraphicSpecularColor=[0.5 0.5 0.5 1.0]  GraphicVisPropType=SimpleVisualProperties
  PS-Simulink Converter1 : nesl_utility/PS-Simulink Converter  PhysicalDomain=network_engine_domain  SubClassName=ps_output  LeftPortType=input  RightPortType=output  PseudoPeriodic=off  Frequencies=[]  Unit=inherit  AffineConversion=off
      settings: SourceProductBaseCode=PW,SS
  PS-Simulink Converter14 : nesl_utility/PS-Simulink Converter  PhysicalDomain=network_engine_domain  SubClassName=ps_output  LeftPortType=input  RightPortType=output  PseudoPeriodic=off  Frequencies=[]  Unit=inherit  AffineConversion=off
      settings: SourceProductBaseCode=PW,SS
  PS-Simulink Converter2 : nesl_utility/PS-Simulink Converter  PhysicalDomain=network_engine_domain  SubClassName=ps_output  LeftPortType=input  RightPortType=output  PseudoPeriodic=off  Frequencies=[]  Unit=inherit  AffineConversion=off
      settings: SourceProductBaseCode=PW,SS
  Rectangular Joint : sm_lib/Joints/Rectangular Joint  JointMode=Normal  SenseConstraintForce=off  SenseConstraintForceX=off  SenseConstraintForceY=off  SenseConstraintForceZ=off  SenseConstraintTorque=off  SenseConstraintTorqueX=off  SenseConstraintTorqueY=off  SenseConstraintTorqueZ=off  SenseTotalForce=off  SenseTotalForceX=off  SenseTotalForceY=off  SenseTotalForceZ=off  SenseTotalTorque=off  SenseTotalTorqueX=off  SenseTotalTorqueY=off  SenseTotalTorqueZ=off  CompositeWrenchDir=FollowerOnBase  CompositeWrenchFrame=BaseFrame  PxEquilibriumPosition=0  PxEquilibriumPositionUnits=m  PxSpringStiffness=0  PxSpringStiffnessUnits=N/m  PxDampingCoefficient=0  PxDampingCoefficientUnits=N/(m/s)  PxTorqueActuationMode=ComputedTorque  PxMotionActuationMode=InputMotion  PxSensePosition=off  PxSenseVelocity=off  PxSenseAcceleration=off  PxSenseTorqueForce=off  PxSenseLowerLimitTorqueForce=off  PxSenseUpperLimitTorqueForce=off  PxLowerLimitSpecify=off  PxLowerLimitBound=-1  PxLowerLimitBoundUnits=m  PxLowerLimitStiffness=1e6  PxLowerLimitStiffnessUnits=N/m  PxLowerLimitDamping=1e3  PxLowerLimitDampingUnits=N/(m/s)  PxLowerLimitTransitionRegionWidth=1e-4  PxLowerLimitTransitionRegionWidthUnits=m  PxUpperLimitSpecify=off  PxUpperLimitBound=1  PxUpperLimitBoundUnits=m  PxUpperLimitStiffness=1e6  PxUpperLimitStiffnessUnits=N/m  PxUpperLimitDamping=1e3  PxUpperLimitDampingUnits=N/(m/s)  PxUpperLimitTransitionRegionWidth=1e-4  PxUpperLimitTransitionRegionWidthUnits=m  PxPositionTargetSpecify=off  PxPositionTargetPriority=High  PxPositionTargetValue=0  PxPositionTargetValueUnits=m  PxVelocityTargetSpecify=off  PxVelocityTargetPriority=High  PxVelocityTargetValue=0  PxVelocityTargetValueUnits=m/s  PyEquilibriumPosition=0  PyEquilibriumPositionUnits=m  PySpringStiffness=0  PySpringStiffnessUnits=N/m  PyDampingCoefficient=0  PyDampingCoefficientUnits=N/(m/s)  PyTorqueActuationMode=ComputedTorque  PyMotionActuationMode=InputMotion  PySensePosition=off  PySenseVelocity=off  PySenseAcceleration=off  PySenseTorqueForce=off  PySenseLowerLimitTorqueForce=off  PySenseUpperLimitTorqueForce=off  PyLowerLimitSpecify=off  PyLowerLimitBound=-1  PyLowerLimitBoundUnits=m  PyLowerLimitStiffness=1e6  PyLowerLimitStiffnessUnits=N/m  PyLowerLimitDamping=1e3  PyLowerLimitDampingUnits=N/(m/s)  PyLowerLimitTransitionRegionWidth=1e-4  PyLowerLimitTransitionRegionWidthUnits=m  PyUpperLimitSpecify=off  PyUpperLimitBound=1  PyUpperLimitBoundUnits=m  PyUpperLimitStiffness=1e6  PyUpperLimitStiffnessUnits=N/m  PyUpperLimitDamping=1e3  PyUpperLimitDampingUnits=N/(m/s)  PyUpperLimitTransitionRegionWidth=1e-4  PyUpperLimitTransitionRegionWidthUnits=m  PyPositionTargetSpecify=off  PyPositionTargetPriority=High  PyPositionTargetValue=0  PyPositionTargetValueUnits=m  PyVelocityTargetSpecify=off  PyVelocityTargetPriority=High  PyVelocityTargetValue=0  PyVelocityTargetValueUnits=m/s
  Revolute Joint : sm_lib/Joints/Revolute Joint  JointMode=Normal  SenseConstraintForce=off  SenseConstraintForceX=off  SenseConstraintForceY=off  SenseConstraintForceZ=off  SenseConstraintTorque=off  SenseConstraintTorqueX=off  SenseConstraintTorqueY=off  SenseConstraintTorqueZ=off  SenseTotalForce=off  SenseTotalForceX=off  SenseTotalForceY=off  SenseTotalForceZ=off  SenseTotalTorque=off  SenseTotalTorqueX=off  SenseTotalTorqueY=off  SenseTotalTorqueZ=off  CompositeWrenchDir=FollowerOnBase  CompositeWrenchFrame=BaseFrame  EquilibriumPosition=0  EquilibriumPositionUnits=deg  SpringStiffness=stif_rot  SpringStiffnessUnits=N*m/rad  DampingCoefficient=damp_rot  DampingCoefficientUnits=N*m/(rad/s)  TorqueActuationMode=NoTorque  MotionActuationMode=ComputedMotion  SensePosition=on  SenseVelocity=on  SenseAcceleration=on  SenseTorqueForce=off  SenseLowerLimitTorqueForce=off  SenseUpperLimitTorqueForce=off  LowerLimitSpecify=on  LowerLimitBound=-45  LowerLimitBoundUnits=deg  LowerLimitStiffness=stif_m  LowerLimitStiffnessUnits=N*m/rad  LowerLimitDamping=damp_m  LowerLimitDampingUnits=N*m/(rad/s)  LowerLimitTransitionRegionWidth=0.1  LowerLimitTransitionRegionWidthUnits=deg  UpperLimitSpecify=on  UpperLimitBound=45  UpperLimitBoundUnits=deg  UpperLimitStiffness=stif_m  UpperLimitStiffnessUnits=N*m/rad  UpperLimitDamping=damp_m  UpperLimitDampingUnits=N*m/(rad/s)  UpperLimitTransitionRegionWidth=0.1  UpperLimitTransitionRegionWidthUnits=deg  PositionTargetSpecify=off  PositionTargetPriority=High  PositionTargetValue=20  PositionTargetValueUnits=deg  VelocityTargetSpecify=off  VelocityTargetPriority=High  VelocityTargetValue=0  VelocityTargetValueUnits=deg/s
  Simulink-PS Converter : nesl_utility/Simulink-PS Converter  PhysicalDomain=network_engine_domain  SubClassName=ps_input  LeftPortType=input  RightPortType=output  PseudoPeriodic=off  Frequencies=[]  NoiseDistribution=none  NoiseParameters=[]  Unit=1  AffineConversion=off  FilteringAndDerivatives=provide  SimscapeFilterOrder=1  InputFilterTimeConstant=0.001  UdotUserProvided=0
      settings: SourceProductBaseCode=PW,SS
  Simulink-PS Converter1 : nesl_utility/Simulink-PS Converter  PhysicalDomain=network_engine_domain  SubClassName=ps_input  LeftPortType=input  RightPortType=output  PseudoPeriodic=off  Frequencies=[]  NoiseDistribution=none  NoiseParameters=[]  Unit=1  AffineConversion=off  FilteringAndDerivatives=provide  SimscapeFilterOrder=1  InputFilterTimeConstant=0.001  UdotUserProvided=0
      settings: SourceProductBaseCode=PW,SS
  Simulink-PS Converter2 : nesl_utility/Simulink-PS Converter  PhysicalDomain=network_engine_domain  SubClassName=ps_input  LeftPortType=input  RightPortType=output  PseudoPeriodic=off  Frequencies=[]  NoiseDistribution=none  NoiseParameters=[]  Unit=1  AffineConversion=off  FilteringAndDerivatives=filter  SimscapeFilterOrder=2  InputFilterTimeConstant=0.001  UdotUserProvided=0
      settings: SourceProductBaseCode=PW,SS
  Simulink-PS Converter3 : nesl_utility/Simulink-PS Converter  PhysicalDomain=network_engine_domain  SubClassName=ps_input  LeftPortType=input  RightPortType=output  PseudoPeriodic=off  Frequencies=[]  NoiseDistribution=none  NoiseParameters=[]  Unit=1  AffineConversion=off  FilteringAndDerivatives=provide  SimscapeFilterOrder=1  InputFilterTimeConstant=0.001  UdotUserProvided=0
      settings: SourceProductBaseCode=PW,SS
  Subsystem1 : Subsystem
  Terminator : Terminator
  Unit Delay : UnitDelay  InitialCondition=-0.51*c_bar  SampleTime=-1  HasFrameUpgradeWarning=on
  left aero force and moment : MATLAB Function  TreatAsAtomicUnit=on
  xy in plane : sm_lib/Frames and Transforms/Rigid Transform  TranslationMethod=None  TranslationStandardOffset=0  TranslationLengthUnit=m  TranslationStandardAxis=+Z  TranslationCartesianOffset=[0 0 0]  TranslationROffset=0  TranslationROffsetUnits=m  TranslationZOffset=0  TranslationZOffsetUnits=m  TranslationThetaOffset=0  TranslationThetaOffsetUnits=deg  RotationMethod=RotationMatrix  RotationAngleUnits=deg  RotationStandardAxis=+Z  RotationAngle=0.0  RotationArbitraryAxis=[0 0 1]  FollAlignAxisA=+X  BaseAlignAxisA=+Y  FollAlignAxisB=+Y  BaseAlignAxisB=+Z  RotationSequenceAxes=FollowerAxes  RotationSequence=XYX  RotationSequenceAngles=[0 0 0]  RotationSequenceAnglesUnits=deg  RotationMatrix=[0 0 1; 0 -1 0; 1 0 0]
  W : PMIOPort  Side=Left
  WT : PMIOPort  Port=2  Side=Left
  CP : PMIOPort  Port=3  Side=Right
  Out Bus Element2 : Outport  PortName=left_rot  Element=b
  Out Bus Element1 : Outport  PortName=left_rot  Element=w
  Out Bus Element7 : Outport  PortName=left_rot  Element=q
  wires:
  PS-Simulink Converter14/1 -> [theta_l]
  PS-Simulink Converter1/1 -> [theta_dot_l]
  PS-Simulink Converter2/1 -> [theta_ddot_l]
  [theta_ddot_l] -> Out Bus Element2/1
  AoA/1(alpha) -> left aero force and moment/2(alpha)
  Subsystem1/1(le0) -> left aero force and moment/1(le0), AoA/1(le0)
  [theta_l] -> AoA/2(rot), Out Bus Element7/1
  [theta_dot_l] -> left aero force and moment/3(rot_dot), Out Bus Element1/1
  [r_cp] -> Simulink-PS Converter3/1
  [d_cp] -> Simulink-PS Converter2/1
  [M_rd] -> Simulink-PS Converter1/1
  [F_N] -> Simulink-PS Converter/1
  Constant/1 -> [r_cp]
  left aero force and moment/2(M_rd) -> [M_rd]
  left aero force and moment/1(F_N) -> [F_N]
  left aero force and moment/4(d_cp) -> Unit Delay/1
  Unit Delay/1 -> [d_cp]
  left aero force and moment/3(M_ae) -> Terminator/1
  connections:
  External Force and Torque1/RConn1 -- xy in plane/LConn1 -- Revolute Joint/RConn1
  Revolute Joint/RConn2 -- PS-Simulink Converter14/LConn1
  Revolute Joint/RConn3 -- PS-Simulink Converter1/LConn1
  Rectangular Joint/LConn1 -- Left Wing/RConn1 -- LWing/RConn1 -- xy in plane/RConn1
  Simulink-PS Converter/RConn1 -- External Force and Torque/LConn2
  Simulink-PS Converter1/RConn1 -- External Force and Torque1/LConn1
  CP/RConn1 -- External Force and Torque/RConn1 -- Graphic/RConn1 -- Rectangular Joint/RConn1
  Revolute Joint/RConn4 -- PS-Simulink Converter2/LConn1
  WT/RConn1 -- Subsystem1/LConn2 -- Revolute Joint/LConn1
  W/RConn1 -- Subsystem1/LConn1
  Simulink-PS Converter2/RConn1 -- Rectangular Joint/LConn3
  Simulink-PS Converter3/RConn1 -- Rectangular Joint/LConn2

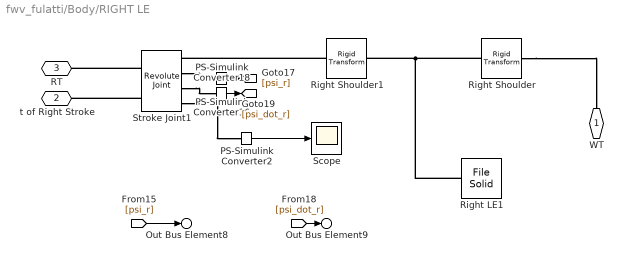
== system fwv_fulatti/Body/RIGHT LE ==
  PS-Simulink Converter16 : nesl_utility/PS-Simulink Converter  PhysicalDomain=network_engine_domain  SubClassName=ps_output  LeftPortType=input  RightPortType=output  PseudoPeriodic=off  Frequencies=[]  Unit=inherit  AffineConversion=off
      settings: SourceProductBaseCode=PW,SS
  PS-Simulink Converter18 : nesl_utility/PS-Simulink Converter  PhysicalDomain=network_engine_domain  SubClassName=ps_output  LeftPortType=input  RightPortType=output  PseudoPeriodic=off  Frequencies=[]  Unit=inherit  AffineConversion=off
      settings: SourceProductBaseCode=PW,SS
  PS-Simulink Converter2 : nesl_utility/PS-Simulink Converter  PhysicalDomain=network_engine_domain  SubClassName=ps_output  LeftPortType=input  RightPortType=output  PseudoPeriodic=off  Frequencies=[]  Unit=inherit  AffineConversion=off
      settings: SourceProductBaseCode=PW,SS
  Right LE1 : sm_lib/Body Elements/File Solid  ExtGeomFileName=meshes/right_LE.step  UnitType=FromFile  ExtGeomFileUnits=m  StepReaderType=HEX  ExportConvexHullGeometry=off  InertiaType=Custom  Mass=1  MassUnits=g  CenterOfMass=[0 -0.0453 0.0239]  CenterOfMassUnits=m  MomentsOfInertia=[3.2e-06, 7.22e-07, 2.48e-06]  MomentsOfInertiaUnits=kg*m^2  ProductsOfInertia=[7.2975e-07 0 0]  ProductsOfInertiaUnits=kg*m^2  BasedOnType=Mass  Density=800  DensityUnits=kg/m^3  DoExposeReferenceFrame=on  SerializedFrames=<Frames/>  GraphicType=FromGeometry  MarkerShape=Sphere  MarkerSize=10  GraphicVisPropType=SimpleVisualProperties  GraphicDiffuseColor=[0.5 0.5 0.5]  GraphicSpecularColor=[0.5 0.5 0.5 1.0]  GraphicAmbientColor=[0.15 0.15 0.15 1.0]  GraphicEmissiveColor=[0.0 0.0 0.0 1.0]  GraphicShininess=75  GraphicOpacity=1.0
  Right Shoulder : sm_lib/Frames and Transforms/Rigid Transform  TranslationMethod=Cartesian  TranslationStandardOffset=0  TranslationLengthUnit=cm  TranslationStandardAxis=+Z  TranslationCartesianOffset=[0 -1 4]  TranslationROffset=0  TranslationROffsetUnits=m  TranslationZOffset=0  TranslationZOffsetUnits=m  TranslationThetaOffset=0  TranslationThetaOffsetUnits=deg  RotationMethod=StandardAxis  RotationAngleUnits=deg  RotationStandardAxis=+X  RotationAngle=-90  RotationArbitraryAxis=[0 0 1]  FollAlignAxisA=+X  BaseAlignAxisA=+Y  FollAlignAxisB=+Y  BaseAlignAxisB=+Z  RotationSequenceAxes=FollowerAxes  RotationSequence=XYX  RotationSequenceAngles=[0 0 0]  RotationSequenceAnglesUnits=deg  RotationMatrix=[0 1 0; 0 0 1; 1 0 0]
  Right Shoulder1 : sm_lib/Frames and Transforms/Rigid Transform  TranslationMethod=None  TranslationStandardOffset=0  TranslationLengthUnit=cm  TranslationStandardAxis=+Z  TranslationCartesianOffset=[0 -1 4]  TranslationROffset=0  TranslationROffsetUnits=m  TranslationZOffset=0  TranslationZOffsetUnits=m  TranslationThetaOffset=0  TranslationThetaOffsetUnits=deg  RotationMethod=StandardAxis  RotationAngleUnits=deg  RotationStandardAxis=+X  RotationAngle=180  RotationArbitraryAxis=[0 0 1]  FollAlignAxisA=+X  BaseAlignAxisA=+Y  FollAlignAxisB=+Y  BaseAlignAxisB=+Z  RotationSequenceAxes=FollowerAxes  RotationSequence=XYX  RotationSequenceAngles=[0 0 0]  RotationSequenceAnglesUnits=deg  RotationMatrix=[0 1 0; 0 0 1; 1 0 0]
  Scope : Scope
  Stroke Joint1 : sm_lib/Joints/Revolute Joint  JointMode=Normal  SenseConstraintForce=off  SenseConstraintForceX=off  SenseConstraintForceY=off  SenseConstraintForceZ=off  SenseConstraintTorque=off  SenseConstraintTorqueX=off  SenseConstraintTorqueY=off  SenseConstraintTorqueZ=off  SenseTotalForce=on  SenseTotalForceX=off  SenseTotalForceY=off  SenseTotalForceZ=off  SenseTotalTorque=off  SenseTotalTorqueX=off  SenseTotalTorqueY=off  SenseTotalTorqueZ=off  CompositeWrenchDir=FollowerOnBase  CompositeWrenchFrame=BaseFrame  EquilibriumPosition=0  EquilibriumPositionUnits=deg  SpringStiffness=stif_stk  SpringStiffnessUnits=N*m/rad  DampingCoefficient=0  DampingCoefficientUnits=N*m/(rad/s)  TorqueActuationMode=ComputedTorque  MotionActuationMode=InputMotion  SensePosition=on  SenseVelocity=on  SenseAcceleration=off  SenseTorqueForce=off  SenseLowerLimitTorqueForce=off  SenseUpperLimitTorqueForce=off  LowerLimitSpecify=on  LowerLimitBound=-90  LowerLimitBoundUnits=deg  LowerLimitStiffness=1e6  LowerLimitStiffnessUnits=N*m/rad  LowerLimitDamping=1e3  LowerLimitDampingUnits=N*m/(rad/s)  LowerLimitTransitionRegionWidth=0.1  LowerLimitTransitionRegionWidthUnits=deg  UpperLimitSpecify=on  UpperLimitBound=90  UpperLimitBoundUnits=deg  UpperLimitStiffness=1e6  UpperLimitStiffnessUnits=N*m/rad  UpperLimitDamping=1e3  UpperLimitDampingUnits=N*m/(rad/s)  UpperLimitTransitionRegionWidth=0.1  UpperLimitTransitionRegionWidthUnits=deg  PositionTargetSpecify=on  PositionTargetPriority=High  PositionTargetValue=30  PositionTargetValueUnits=deg  VelocityTargetSpecify=off  VelocityTargetPriority=High  VelocityTargetValue=0  VelocityTargetValueUnits=deg/s
  WT : PMIOPort  Side=Left
  t of Right Stroke : PMIOPort  Port=2  Side=Right
  RT : PMIOPort  Port=3  Side=Right
  Out Bus Element8 : Outport  PortName=right_stk  Element=q
  Out Bus Element9 : Outport  PortName=right_stk  Element=w
  wires:
  PS-Simulink Converter18/1 -> [psi_dot_r]
  PS-Simulink Converter2/1 -> Scope/1
  PS-Simulink Converter16/1 -> [psi_r]
  [psi_dot_r] -> Out Bus Element9/1
  [psi_r] -> Out Bus Element8/1
  connections:
  Stroke Joint1/RConn2 -- PS-Simulink Converter16/LConn1
  Stroke Joint1/LConn1 -- RT/RConn1
  Right Shoulder1/LConn1 -- Stroke Joint1/RConn1
  Stroke Joint1/RConn4 -- PS-Simulink Converter2/LConn1
  Stroke Joint1/RConn3 -- PS-Simulink Converter18/LConn1
  Stroke Joint1/LConn2 -- t of Right Stroke/RConn1
  Right Shoulder/RConn1 -- WT/RConn1
  Right Shoulder/LConn1 -- Right LE1/RConn1 -- Right Shoulder1/RConn1
